simulink library "ad_mtx_scalar"  (R2017a)
settings: Solver=VariableStepAuto  StartTime=0.0  StopTime=10.0  RelTol=1e-3
libraries: autodiff x4
settings Model: Creator=eruffaldi  LastModifiedBy=eruffaldi

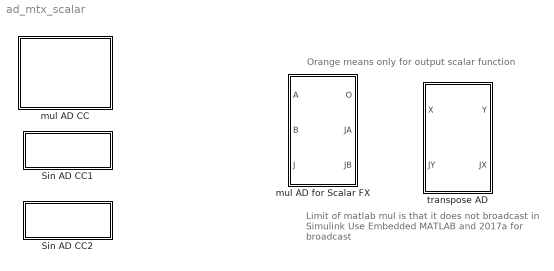
== system ad_mtx_scalar ==
  note: Orange means only for output scalar function
  note: Limit of matlab mul is that it does not broadcast
      | in Simulink
      |
      | Use Embedded MATLAB and 2017a for broadcast
  Sin AD CC1 : Subsystem
      mask Display: disp('inv(x)');
  Sin AD CC2 : Subsystem
      mask Display: disp('transpose(x)');
  mul AD CC : Subsystem
  mul AD for Scalar FX : Subsystem
  transpose AD : Subsystem

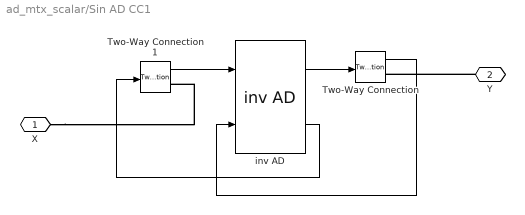
== system ad_mtx_scalar/Sin AD CC1 ==
  Two-Way Connection : TwoWayConnection
  Two-Way Connection1 : TwoWayConnection
  inv AD : autodiff/inv AD
      settings: SourceProductName=AutoDiff
  X : PMIOPort  Port=1  Side=Left
  Y : PMIOPort  Port=2  Side=Right
  wires:
  inv AD/2 -> Two-Way Connection1/1
  Two-Way Connection1/1 -> inv AD/1
  Two-Way Connection/1 -> inv AD/2
  inv AD/1 -> Two-Way Connection/1
  connections:
  Y/RConn1 -- Two-Way Connection/RConn1
  X/RConn1 -- Two-Way Connection1/RConn1

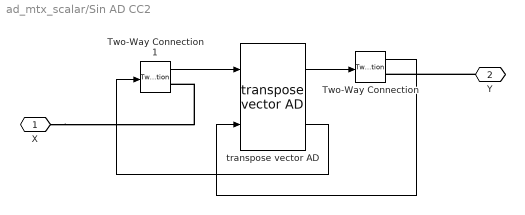
== system ad_mtx_scalar/Sin AD CC2 ==
  Two-Way Connection : TwoWayConnection
  Two-Way Connection1 : TwoWayConnection
  transpose vector AD : autodiff/transpose vector AD
      settings: SourceProductName=AutoDiff
  X : PMIOPort  Port=1  Side=Left
  Y : PMIOPort  Port=2  Side=Right
  wires:
  transpose vector AD/1 -> Two-Way Connection/1
  Two-Way Connection/1 -> transpose vector AD/2
  Two-Way Connection1/1 -> transpose vector AD/1
  transpose vector AD/2 -> Two-Way Connection1/1
  connections:
  X/RConn1 -- Two-Way Connection1/RConn1
  Y/RConn1 -- Two-Way Connection/RConn1

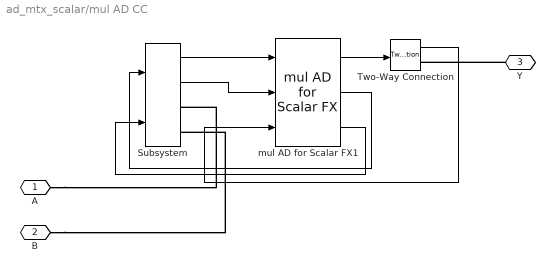
== system ad_mtx_scalar/mul AD CC ==
  Subsystem : autodiff/Plus AD CC/Subsystem
      settings: SourceProductName=AutoDiff
  Two-Way Connection : TwoWayConnection
  mul AD for Scalar FX1 : autodiff/mul AD for Scalar FX
      settings: SourceProductName=AutoDiff
  A : PMIOPort  Port=1  Side=Left
  B : PMIOPort  Port=2  Side=Left
  Y : PMIOPort  Port=3  Side=Right
  wires:
  Subsystem/1 -> mul AD for Scalar FX1/1
  mul AD for Scalar FX1/2 -> Subsystem/1
  Two-Way Connection/1 -> mul AD for Scalar FX1/3
  Subsystem/2 -> mul AD for Scalar FX1/2
  mul AD for Scalar FX1/3 -> Subsystem/2
  mul AD for Scalar FX1/1 -> Two-Way Connection/1
  connections:
  B/RConn1 -- Subsystem/RConn2
  A/RConn1 -- Subsystem/RConn1
  Y/RConn1 -- Two-Way Connection/RConn1

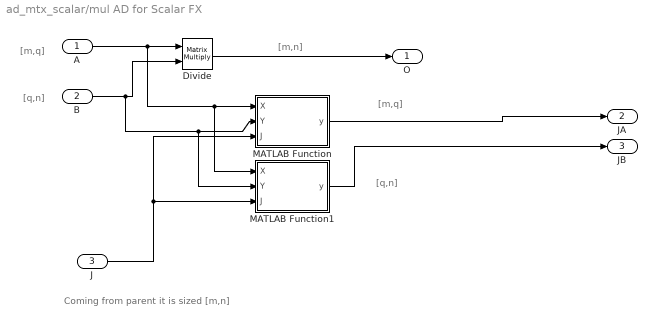
== system ad_mtx_scalar/mul AD for Scalar FX ==
  note: [q,n]
  note: [m,q]
  note: [m,n]
  note: [q,n]
  note: [m,q]
  note: Coming from parent it is sized [m,n]
  A : Inport
  B : Inport  Port=2
  J : Inport  Port=3
  Divide : Product  Inputs=**  Multiplication=Matrix(*)
  MATLAB Function : MATLAB Function  TreatAsAtomicUnit=on
  MATLAB Function1 : MATLAB Function  TreatAsAtomicUnit=on
  O : Outport
  JA : Outport  Port=2
  JB : Outport  Port=3
  wires:
  Divide/1 -> O/1
  A/1 -> MATLAB Function1/1(X), MATLAB Function/1(X), Divide/1
  MATLAB Function1/1(y) -> JB/1
  MATLAB Function/1(y) -> JA/1
  B/1 -> MATLAB Function1/2(Y), MATLAB Function/2(Y), Divide/2
  J/1 -> MATLAB Function1/3(J), MATLAB Function/3(J)

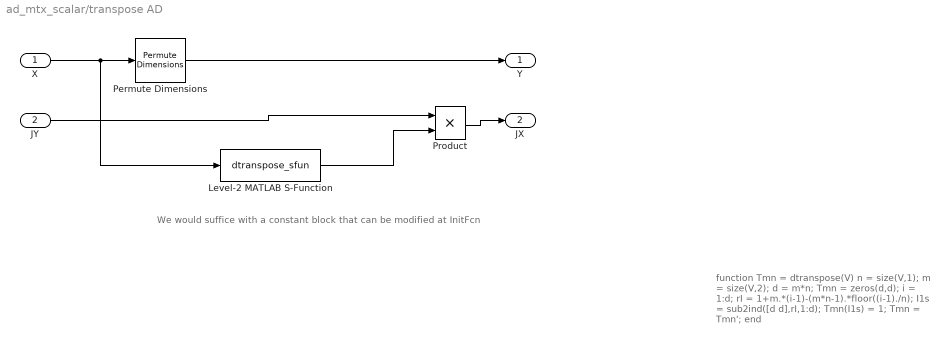
== system ad_mtx_scalar/transpose AD ==
  note: We would suffice with a constant block that can be modified at InitFcn
  note: function Tmn = dtranspose(V)
      |             n = size(V,1);
      |             m = size(V,2);
      |             d = m*n;
      |             Tmn = zeros(d,d);
      |
      |             i = 1:d;
      |             rI = 1+m.*(i-1)-(m*n-1).*floor((i-1)./n);
      |             I1s = sub2ind([d d],rI,1:d);
      |             Tmn(I1s) = 1;
      |             Tmn = Tmn';
      |         end
  X : Inport
  JY : Inport  Port=2
  Level-2 MATLAB S-Function : M-S-Function  FunctionName=dtranspose_sfun
  Permute Dimensions : PermuteDimensions
  Product : Product
  Y : Outport
  JX : Outport  Port=2
  wires:
  Permute Dimensions/1 -> Y/1
  X/1 -> Level-2 MATLAB S-Function/1, Permute Dimensions/1
  Product/1 -> JX/1
  Level-2 MATLAB S-Function/1 -> Product/2
  JY/1 -> Product/1

== matlab function ad_mtx_scalar/mul AD for Scalar FX/MATLAB Function1 ==
  data: X input; y output; Y input; J input
function y = fcn(X,Y,J)
%#codegen

y = repmat(reshape(sum(X,1),size(X,2),1),1,size(Y,2));
if length(J) == 1
    y = J*y;
else
    y = repmat(sum(J,1),size(Y,1),1).*y;
end

== matlab function ad_mtx_scalar/mul AD for Scalar FX/MATLAB Function ==
  data: X input; y output; Y input; J input
function y = fcn(X,Y,J)
%#codegen

y = repmat(reshape(sum(Y,2),1,size(Y,1)),size(X,1),1);
if length(J) == 1
    y = J*y;
else
    y = repmat(sum(J,2),1,size(X,2)).*y;
end
